simulink model "Week3_Problem1"  (R2020b)
settings: Solver=VariableStepAuto  StartTime=0.0  StopTime=10.0  RelTol=1e-3
settings Model: Creator=ASUS  LastModifiedBy=ASUS

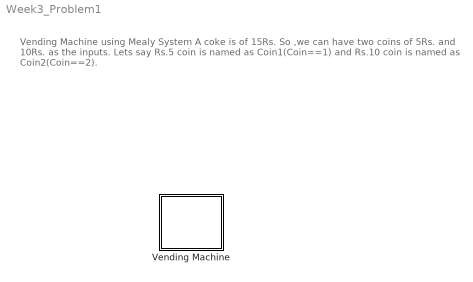
== system Week3_Problem1 ==
  note: Vending Machine using Mealy System
      |
      | A coke is of 15Rs. So ,we can have two coins of 5Rs. and 10Rs. as the inputs.
      | Lets say Rs.5 coin is named as Coin1(Coin==1) and Rs.10 coin is named as Coin2(Coin==2).
  Vending Machine : Stateflow chart  TreatAsAtomicUnit=on

== stateflow chart Week3_Problem1/Vending Machine ==
  state zero_Rs
  state Five_Rs
  state Ten_Rs
  (default) -> zero_Rs
